simulink model "control_6dof"  (R2024b)
settings: configuration reference "prj_default_config" (kept outside this file)
values from neighbouring files (symbols this model uses):
  CONTROL_PARAM = Simulink.Parameter(CONTROL_PARAM_VALUE)    [control_init.m]
undefined symbols (not defined in the file or in its folder): CONTROL_CONST
libraries: mqlib x3
settings Model: Creator=yangyu  LastModifiedBy=yangyu
settings ConfigSetRef: SourceName=prj_default_config  SourceLocation=Base Workspace

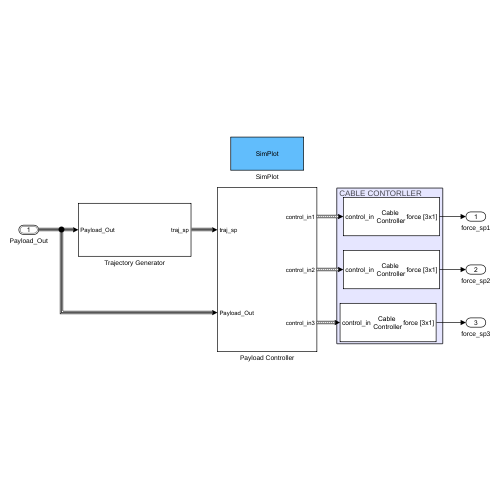
[thumbnail: Simulink's stored preview of the top-level diagram]
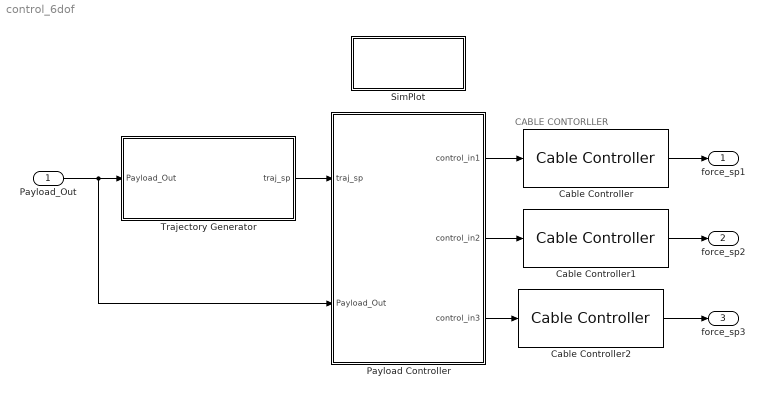
== system control_6dof ==
  note: CABLE CONTORLLER
  Payload_Out : Inport  OutDataTypeStr=Bus: Payload_Out_Bus
  Cable Controller : mqlib/Cable Controller  Kq=CONTROL_PARAM.KQ  Kw=CONTROL_PARAM.KW  mi=CONTROL_PARAM.MASS_UAV  li=CONTROL_PARAM.CABLE_LEN
  Cable Controller1 : mqlib/Cable Controller  Kq=CONTROL_PARAM.KQ  Kw=CONTROL_PARAM.KW  mi=CONTROL_PARAM.MASS_UAV  li=CONTROL_PARAM.CABLE_LEN
  Cable Controller2 : mqlib/Cable Controller  Kq=CONTROL_PARAM.KQ  Kw=CONTROL_PARAM.KW  mi=CONTROL_PARAM.MASS_UAV  li=CONTROL_PARAM.CABLE_LEN
  Payload Controller : Subsystem
  SimPlot : Subsystem
      settings: OpenFcn=run('simplot.m');
      mask Display: disp('SimPlot');
  Trajectory Generator : Subsystem
  force_sp1 : Outport  PortDimensions=3
  force_sp2 : Outport  Port=2  PortDimensions=3
  force_sp3 : Outport  Port=3  PortDimensions=3
  wires:
  Trajectory Generator/1(traj_sp) -> Payload Controller/1(traj_sp)
  Payload_Out/1 -> Payload Controller/2(Payload_Out), Trajectory Generator/1(Payload_Out)
  Cable Controller/1 -> force_sp1/1
  Cable Controller1/1 -> force_sp2/1
  Cable Controller2/1 -> force_sp3/1
  Payload Controller/1(control_in1) -> Cable Controller/1
  Payload Controller/2(control_in2) -> Cable Controller1/1
  Payload Controller/3(control_in3) -> Cable Controller2/1

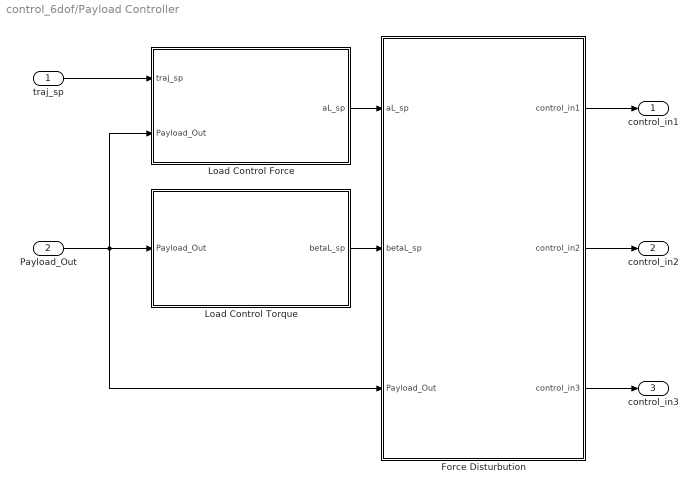
== system control_6dof/Payload Controller ==
  traj_sp : Inport
  Payload_Out : Inport  Port=2
  Force Disturbution : MATLAB Function  TreatAsAtomicUnit=on  mask{rho=CONTROL_PARAM.RHO, mL=CONTROL_PARAM.MASS_LOAD}
  Load Control Force : Subsystem
  Load Control Torque : Subsystem
  control_in1 : Outport
  control_in2 : Outport  Port=2
  control_in3 : Outport  Port=3
  wires:
  traj_sp/1 -> Load Control Force/1(traj_sp)
  Force Disturbution/1(control_in1) -> control_in1/1
  Force Disturbution/2(control_in2) -> control_in2/1
  Force Disturbution/3(control_in3) -> control_in3/1
  Payload_Out/1 -> Force Disturbution/3(Payload_Out), Load Control Force/2(Payload_Out), Load Control Torque/1(Payload_Out)
  Load Control Torque/1(betaL_sp) -> Force Disturbution/2(betaL_sp)
  Load Control Force/1(aL_sp) -> Force Disturbution/1(aL_sp)

== system control_6dof/SimPlot ==

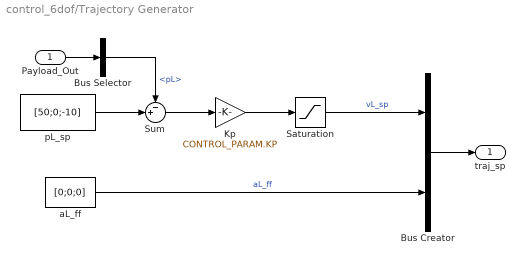
== system control_6dof/Trajectory Generator ==
  Payload_Out : Inport
  Bus Creator : BusCreator  Inputs=2
  Bus Selector : BusSelector  OutputSignals=pL
  Kp : Gain  Gain=CONTROL_PARAM.KP
  Saturation : Saturate  UpperLimit=2  LowerLimit=-2
  Sum : Sum  Inputs=-+|
  aL_ff : Constant  Value=[0;0;0]
  pL_sp : Constant  Value=[50;0;-10]
  traj_sp : Outport
  wires:
  Saturation/1 -> Bus Creator/1  "vL_sp"
  Bus Creator/1 -> traj_sp/1
  pL_sp/1 -> Sum/2
  Payload_Out/1 -> Bus Selector/1
  Bus Selector/1 -> Sum/1  "<pL>"
  Sum/1 -> Kp/1
  Kp/1 -> Saturation/1
  aL_ff/1 -> Bus Creator/2  "aL_ff"

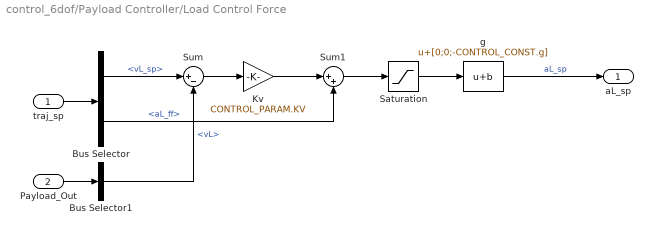
== system control_6dof/Payload Controller/Load Control Force ==
  traj_sp : Inport
  Payload_Out : Inport  Port=2
  Bus Selector : BusSelector  OutputSignals=vL_sp,aL_ff
  Bus Selector1 : BusSelector  OutputSignals=vL
  Kv : Gain  Gain=CONTROL_PARAM.KV
  Saturation : Saturate  UpperLimit=Inf  LowerLimit=-inf
  Sum : Sum  Inputs=|+-
  Sum1 : Sum  Inputs=|++
  g : Bias  Bias=[0;0;-CONTROL_CONST.g]  SaturateOnIntegerOverflow=off
  aL_sp : Outport
  wires:
  g/1 -> aL_sp/1  "aL_sp"
  traj_sp/1 -> Bus Selector/1
  Sum/1 -> Kv/1
  Kv/1 -> Sum1/1
  Bus Selector/1 -> Sum/1  "<vL_sp>"
  Bus Selector1/1 -> Sum/2  "<vL>"
  Saturation/1 -> g/1
  Bus Selector/2 -> Sum1/2  "<aL_ff>"
  Sum1/1 -> Saturation/1
  Payload_Out/1 -> Bus Selector1/1

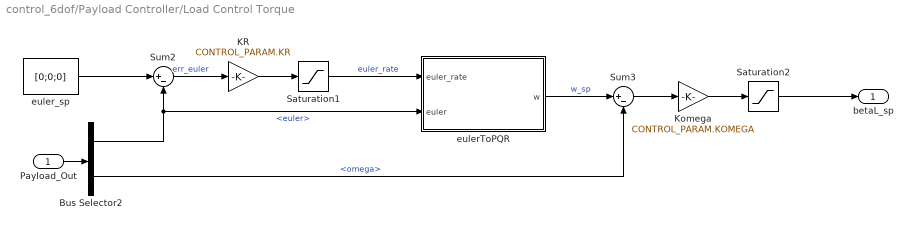
== system control_6dof/Payload Controller/Load Control Torque ==
  Payload_Out : Inport
  Bus Selector2 : BusSelector  OutputSignals=euler,omega
  KR : Gain  Gain=CONTROL_PARAM.KR
  Komega : Gain  Gain=CONTROL_PARAM.KOMEGA
  Saturation1 : Saturate  UpperLimit=inf  LowerLimit=-inf
  Saturation2 : Saturate  UpperLimit=inf  LowerLimit=-inf
  Sum2 : Sum  Inputs=|+-
  Sum3 : Sum  Inputs=|+-
  eulerToPQR : MATLAB Function  TreatAsAtomicUnit=on
  euler_sp : Constant  Value=[0;0;0]
  betaL_sp : Outport
  wires:
  Sum2/1 -> KR/1  "err_euler"
  KR/1 -> Saturation1/1
  Sum3/1 -> Komega/1
  eulerToPQR/1(w) -> Sum3/1  "w_sp"
  Saturation1/1 -> eulerToPQR/1(euler_rate)  "euler_rate"
  Bus Selector2/2 -> Sum3/2  "<omega>"
  Komega/1 -> Saturation2/1
  euler_sp/1 -> Sum2/1
  Saturation2/1 -> betaL_sp/1
  Bus Selector2/1 -> Sum2/2, eulerToPQR/2(euler)  "<euler>"
  Payload_Out/1 -> Bus Selector2/1

== matlab function control_6dof/Payload Controller/Force Disturbution ==
  data: aL_sp input; betaL_sp input; control_in1 output Bus: Control_In_Bus; Payload_Out input Bus: Payload_Out_Bus; rho parameter; control_in2 output Bus: Control_In_Bus; control_in3 output Bus: Control_In_Bus; mL parameter
function [control_in1, control_in2, control_in3] = fcn(aL_sp, betaL_sp, Payload_Out, rho, mL)
RL = eulerToDCM(Payload_Out.euler);
P = [eye(3) eye(3) eye(3); hat_map(rho(:, 1)) hat_map(rho(:, 2)) hat_map(rho(:, 3))];
vu = blkdiag(RL, RL, RL) * pinv(P) * [RL'*aL_sp*mL; betaL_sp];
% persistent vu cnt;
% if isempty(cnt)
%     cnt = 0;
% end
% cnt = cnt + 1;
% if isempty(vu) || cnt == 10
% 
%     cnt = 0;
% end

control_in1.timestamp = uint32(1);
control_in1.vforce = vu(1:3);
control_in1.q_sp = -control_in1.vforce / norm(control_in1.vforce);
control_in1.q = Payload_Out.q_1;
control_in1.w = Payload_Out.w_1;
control_in1.ai_sp = aL_sp + RL * cross(Payload_Out.omega, cross(Payload_Out.omega, rho(:, 1))) - RL * cross(rho(:, 1), betaL_sp);

control_in2.timestamp = uint32(1);
control_in2.vforce = vu(4:6);
control_in2.q_sp = -control_in2.vforce / norm(control_in2.vforce);
control_in2.q = Payload_Out.q_2;
control_in2.w = Payload_Out.w_2;
control_in2.ai_sp = aL_sp + RL * cross(Payload_Out.omega, cross(Payload_Out.omega, rho(:, 2))) - RL * cross(rho(:, 2), betaL_sp);

control_in3.timestamp = uint32(1);
control_in3.vforce = vu(7:9);
control_in3.q_sp = -control_in3.vforce / norm(control_in3.vforce);
control_in3.q = Payload_Out.q_3;
control_in3.w = Payload_Out.w_3;
control_in3.ai_sp = aL_sp + RL * cross(Payload_Out.omega, cross(Payload_Out.omega, rho(:, 3))) - RL * cross(rho(:, 3), betaL_sp);

end

function so3 = hat_map(r3)
    so3 = [0 -r3(3) r3(2); r3(3) 0 -r3(1); -r3(2) r3(1) 0];
end

function R = eulerToDCM(eluer)
    Rx = [1, 0, 0;
          0, cos(eluer(1)), -sin(eluer(1));
          0, sin(eluer(1)), cos(eluer(1))];
    Ry = [cos(eluer(2)), 0, sin(eluer(2));
          0, 1, 0;
          -sin(eluer(2)), 0, cos(eluer(2))];
    Rz = [cos(eluer(3)), -sin(eluer(3)), 0;
          sin(eluer(3)), cos(eluer(3)), 0;
          0, 0, 1];
    R = Rz * Ry * Rx;
end

== matlab function control_6dof/Payload Controller/Load Control Torque/eulerToPQR ==
  data: euler_rate input; euler input; w output
function w = fcn(euler_rate, euler)

    % 计算滚转速率 p
    p = euler_rate(1) + sin(euler(1)) * tan(euler(2)) * euler_rate(2) + cos(euler(1)) * tan(euler(2)) * euler_rate(3);

    % 计算俯仰速率 q
    q = cos(euler(1)) * euler_rate(2) - sin(euler(1)) * euler_rate(3);

    % 计算偏航速率 r
    r = (sin(euler(1)) / cos(euler(2))) * euler_rate(2) + (cos(euler(1)) / cos(euler(2))) * euler_rate(3);

    w = [p, q, r];
end
